simulink subsystem "Odometria"  (R2023b)
settings: Solver=VariableStepAuto  StartTime=0.0  StopTime=10.0  RelTol=1e-3
settings Model: Creator=Antonio  LastModifiedBy=Antonio

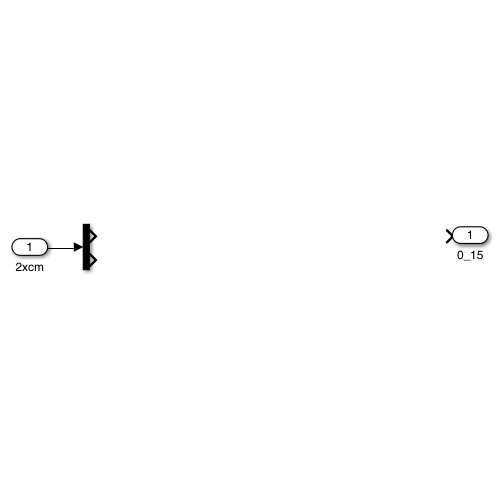
[thumbnail: Simulink's stored preview of the top-level diagram]
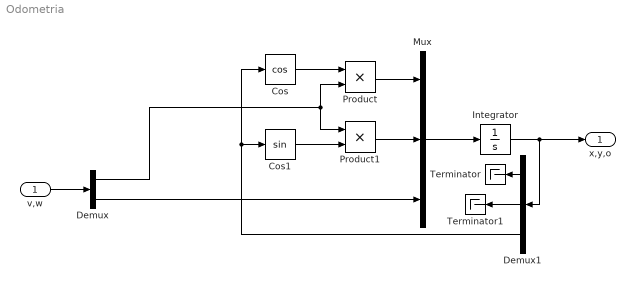
== system Odometria ==
  v,w : Inport
  Cos : Trigonometry  Operator=cos
  Cos1 : Trigonometry
  Demux : Demux  Outputs=2
  Demux1 : Demux  Outputs=3
  Integrator : Integrator
  Mux : Mux  Inputs=3
  Product : Product
  Product1 : Product
  Terminator : Terminator
  Terminator1 : Terminator
  x,y,o : Outport
  wires:
  v,w/1 -> Demux/1
  Cos/1 -> Product/1
  Cos1/1 -> Product1/2
  Integrator/1 -> x,y,o/1, Demux1/1
  Mux/1 -> Integrator/1
  Product/1 -> Mux/1
  Product1/1 -> Mux/2
  Demux/2 -> Mux/3
  Demux1/3 -> Cos1/1, Cos/1
  Demux/1 -> Product/2, Product1/1
  Demux1/1 -> Terminator/1
  Demux1/2 -> Terminator1/1
